simulink model "parte1_eje15_controlPID"  (R2017b)
settings: Solver=VariableStepAuto  StartTime=0.0  StopTime=10.0  RelTol=1e-3
settings Model: Creator=cjuar  LastModifiedBy=cjuar

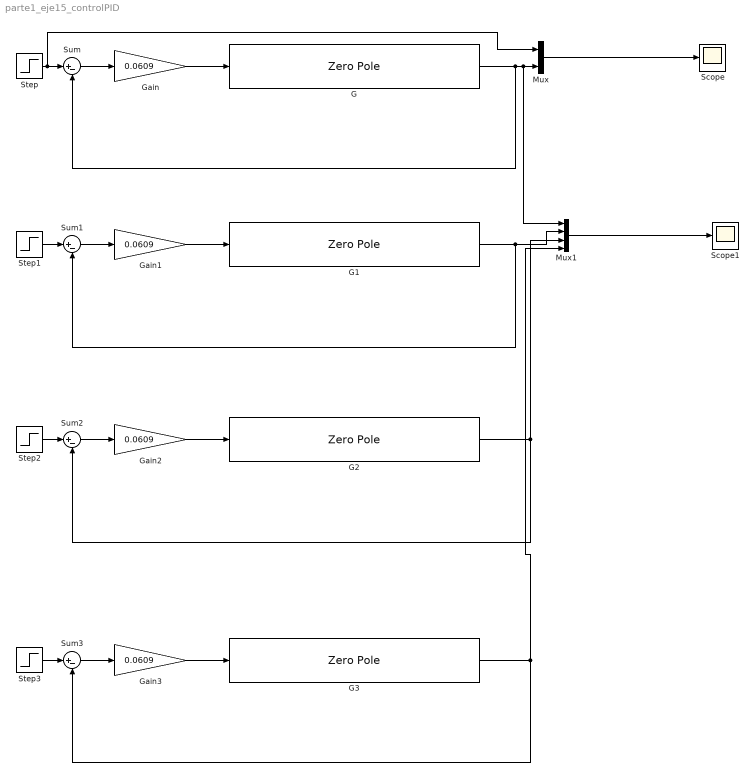
== system parte1_eje15_controlPID ==
  G : ZeroPole  Zeros=[-11.136 -0.1]  Poles=[0 0 -6 -18]  Gain=[1080]
  G1 : ZeroPole  Zeros=[]  Poles=[0 -6 -18]  Gain=[1080]
  G2 : ZeroPole  Zeros=[-11.136 ]  Poles=[0 -6 -18]  Gain=[1080]
  G3 : ZeroPole  Zeros=[-0.1 ]  Poles=[0 0 -6 -18]  Gain=[1080]
  Gain{,1..3} (4 alike) : Gain  Gain=0.0609
  Mux : Mux  Inputs=2
  Mux1 : Mux
  Scope : Scope
  Scope1 : Scope
  Step{,1..3} (4 alike) : Step  SampleTime=0
  Sum{,1..3} (4 alike) : Sum  Inputs=|+-
  wires:
  Gain/1 -> G/1
  Step/1 -> Mux/1, Sum/1
  Sum/1 -> Gain/1
  Mux/1 -> Scope/1
  G/1 -> Mux1/1, Mux/2, Sum/2
  Gain1/1 -> G1/1
  Sum1/1 -> Gain1/1
  G1/1 -> Mux1/2, Sum1/2
  Mux1/1 -> Scope1/1
  Step1/1 -> Sum1/1
  Step2/1 -> Sum2/1
  G2/1 -> Sum2/2, Mux1/3
  Sum2/1 -> Gain2/1
  Gain2/1 -> G2/1
  Gain3/1 -> G3/1
  Sum3/1 -> Gain3/1
  G3/1 -> Mux1/4, Sum3/2
  Step3/1 -> Sum3/1
